simulink model "rlFlyingRobotEnv"  (R2021b)
settings: Solver=VariableStepAuto  StartTime=0.0  StopTime=30  RelTol=1e-3
values from neighbouring files (symbols this model uses):
  theta0 = 0    [main.m]
  Ts = 0.4    [main.m]
  x0 = -15    [main.m]
  y0 = 0    [main.m]
libraries: simulink x3
settings Model: Creator=The MathWorks, Inc.  LastModifiedBy=geek
settings SolverCC: AlgebraicLoopSolver=TrustRegion
settings DataIOCC: ReturnWorkspaceOutputs=off
settings DebuggingCC: SFMachineParentedDataDiag=warning  ArithmeticOperatorsInVariantConditions=warning
settings ModelReferenceCC: ModelReferenceMinAlgLoopOccurrences=on

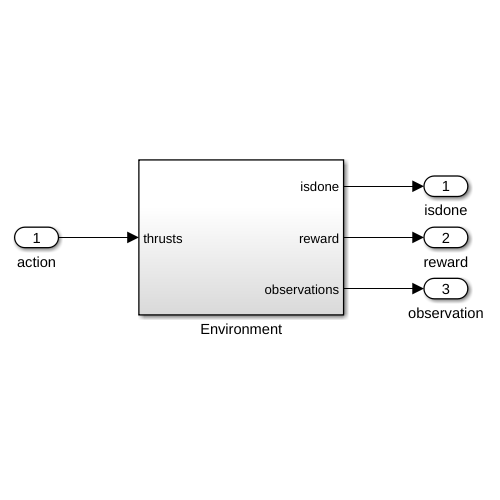
[thumbnail: Simulink's stored preview of the top-level diagram]
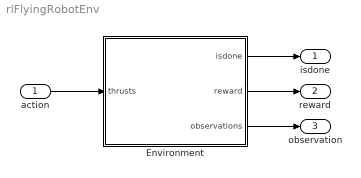
== system rlFlyingRobotEnv ==
  action : Inport
  Environment : Subsystem
  isdone : Outport  VectorParamsAs1DForOutWhenUnconnected=off
  reward : Outport  Port=2  VectorParamsAs1DForOutWhenUnconnected=off
  observation : Outport  Port=3  VectorParamsAs1DForOutWhenUnconnected=off
  wires:
  Environment/3(observations) -> observation/1
  Environment/2(reward) -> reward/1
  Environment/1(isdone) -> isdone/1
  action/1 -> Environment/1(thrusts)

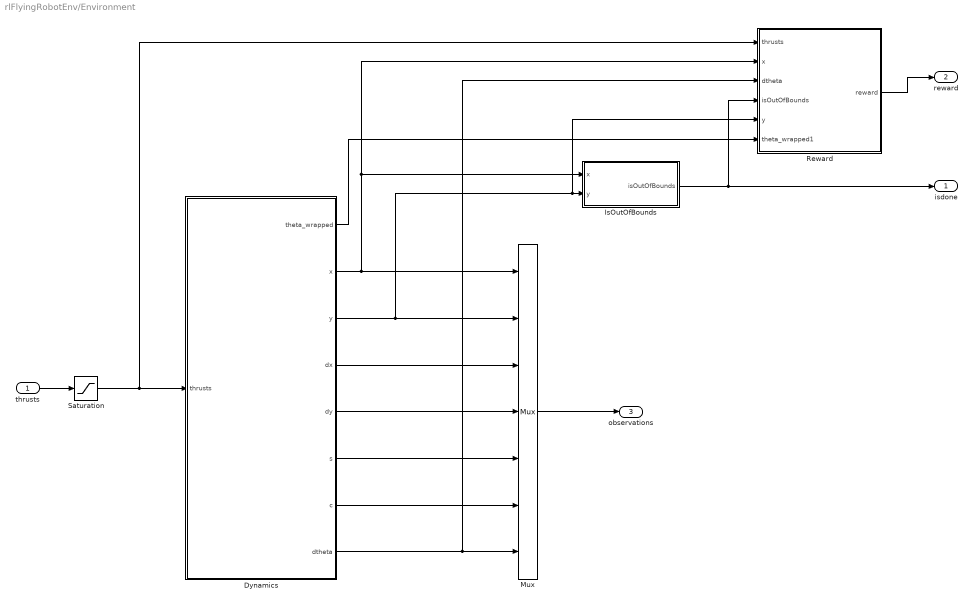
== system rlFlyingRobotEnv/Environment ==
  thrusts : Inport
  Dynamics : Subsystem
  IsOutOfBounds : Subsystem
  Mux : Mux  Inputs=7
  Reward : Subsystem
  Saturation : Saturate  UpperLimit=1  LowerLimit=-1
  isdone : Outport  VectorParamsAs1DForOutWhenUnconnected=off
  reward : Outport  Port=2  VectorParamsAs1DForOutWhenUnconnected=off
  observations : Outport  Port=3  VectorParamsAs1DForOutWhenUnconnected=off
  wires:
  Reward/1(reward) -> reward/1
  IsOutOfBounds/1(isOutOfBounds) -> isdone/1, Reward/4(isOutOfBounds)
  Dynamics/3(y) -> Mux/2, Reward/5(y), IsOutOfBounds/2(y)
  Dynamics/2(x) -> Mux/1, IsOutOfBounds/1(x), Reward/2(x)
  Mux/1 -> observations/1
  Saturation/1 -> Reward/1(thrusts), Dynamics/1(thrusts)
  thrusts/1 -> Saturation/1
  Dynamics/4(dx) -> Mux/3
  Dynamics/5(dy) -> Mux/4
  Dynamics/6(s) -> Mux/5
  Dynamics/7(c) -> Mux/6
  Dynamics/8(dtheta) -> Reward/3(dtheta), Mux/7
  Dynamics/1(theta_wrapped) -> Reward/6(theta_wrapped1)

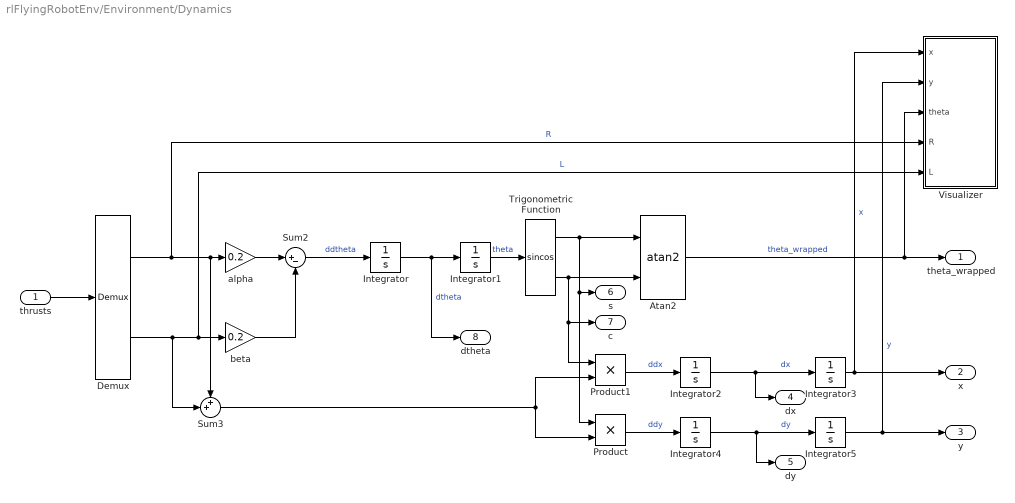
== system rlFlyingRobotEnv/Environment/Dynamics ==
  thrusts : Inport
  Atan2 : Trigonometry  Operator=atan2
  Demux : Demux  Outputs=2
  Integrator : Integrator
  Integrator1 : Integrator  InitialCondition=theta0
  Integrator2 : Integrator
  Integrator3 : Integrator  InitialCondition=x0
  Integrator4 : Integrator
  Integrator5 : Integrator  InitialCondition=y0
  Product : Product
  Product1 : Product
  Sum2 : Sum  Inputs=|+-
  Sum3 : Sum  Inputs=++|
  Trigonometric Function : Trigonometry  Operator=sincos
  Visualizer : Subsystem
  alpha : Gain  Gain=0.2
  beta : Gain  Gain=0.2
  theta_wrapped : Outport  VectorParamsAs1DForOutWhenUnconnected=off
  x : Outport  Port=2  VectorParamsAs1DForOutWhenUnconnected=off
  y : Outport  Port=3  VectorParamsAs1DForOutWhenUnconnected=off
  dx : Outport  Port=4  VectorParamsAs1DForOutWhenUnconnected=off
  dy : Outport  Port=5  VectorParamsAs1DForOutWhenUnconnected=off
  s : Outport  Port=6  VectorParamsAs1DForOutWhenUnconnected=off
  c : Outport  Port=7  VectorParamsAs1DForOutWhenUnconnected=off
  dtheta : Outport  Port=8  VectorParamsAs1DForOutWhenUnconnected=off
  wires:
  Integrator1/1 -> Trigonometric Function/1  "theta"
  Product1/1 -> Integrator2/1  "ddx"
  Integrator2/1 -> dx/1, Integrator3/1  "dx"
  Demux/2 -> Sum3/2, Visualizer/5(L), beta/1  "L"
  Demux/1 -> Visualizer/4(R), Sum3/1, alpha/1  "R"
  Sum3/1 -> Product1/2, Product/2
  Integrator4/1 -> Integrator5/1, dy/1  "dy"
  Trigonometric Function/1 -> s/1, Product/1, Atan2/1
  Trigonometric Function/2 -> Product1/1, c/1, Atan2/2
  Sum2/1 -> Integrator/1  "ddtheta"
  Integrator3/1 -> Visualizer/1(x), x/1  "x"
  Integrator/1 -> dtheta/1, Integrator1/1  "dtheta"
  Product/1 -> Integrator4/1  "ddy"
  Integrator5/1 -> Visualizer/2(y), y/1  "y"
  alpha/1 -> Sum2/1
  beta/1 -> Sum2/2
  thrusts/1 -> Demux/1
  Atan2/1 -> Visualizer/3(theta), theta_wrapped/1  "theta_wrapped"

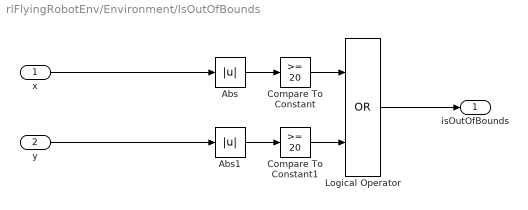
== system rlFlyingRobotEnv/Environment/IsOutOfBounds ==
  x : Inport
  y : Inport  Port=2
  Abs : Abs
  Abs1 : Abs
  Compare To Constant : simulink/Logic and Bit Operations/Compare To Constant  relop=>=  const=20  OutDataTypeStr=boolean
  Compare To Constant1 : simulink/Logic and Bit Operations/Compare To Constant  relop=>=  const=20  OutDataTypeStr=boolean
  Logical Operator : Logic  Operator=OR  AllPortsSameDT=off  OutDataTypeStr=boolean
  isOutOfBounds : Outport  VectorParamsAs1DForOutWhenUnconnected=off
  wires:
  Compare To Constant1/1 -> Logical Operator/2
  Compare To Constant/1 -> Logical Operator/1
  y/1 -> Abs1/1
  Abs/1 -> Compare To Constant/1
  x/1 -> Abs/1
  Abs1/1 -> Compare To Constant1/1
  Logical Operator/1 -> isOutOfBounds/1

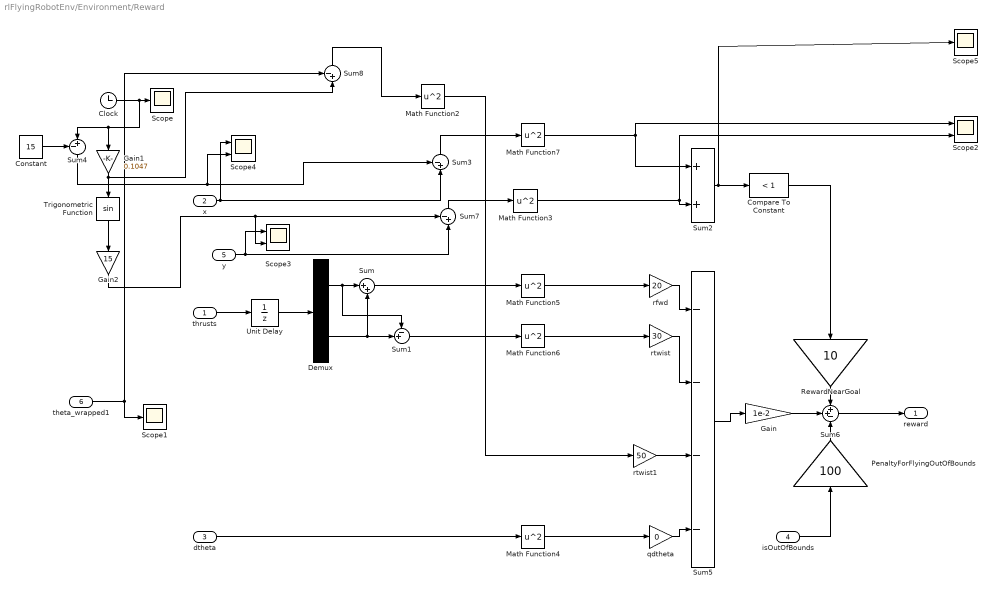
== system rlFlyingRobotEnv/Environment/Reward ==
  thrusts : Inport
  x : Inport  Port=2
  dtheta : Inport  Port=3
  isOutOfBounds : Inport  Port=4
  y : Inport  Port=5
  theta_wrapped1 : Inport  Port=6
  Clock : Clock
      settings: Decimation=30
  Compare To Constant : simulink/Logic and Bit Operations/Compare To Constant  relop=<  const=1  OutDataTypeStr=boolean
  Constant : Constant  Value=15
  Demux : Demux  Outputs=2
  Gain : Gain  Gain=1e-2
  Gain1 : Gain  Gain=0.1047
  Gain2 : Gain  Gain=15
  Math Function{2..7} (6 alike) : Math  Operator=square  SignedPower=on  SaturateOnIntegerOverflow=on
  PenaltyForFlyingOutOfBounds : Gain  Gain=100
  RewardNearGoal : Gain  Gain=10
  Scope : Scope
  Scope1 : Scope
  Scope2 : Scope  NumInputPorts=2
  Scope3 : Scope  NumInputPorts=2
  Scope4 : Scope  NumInputPorts=2
  Scope5 : Scope
  Sum : Sum  Inputs=|++
  Sum{1,3..4,7..8} (5 alike) : Sum  Inputs=-+|
  Sum2 : Sum
  Sum5 : Sum  Inputs=----
  Sum6 : Sum  Inputs=++-
  Trigonometric Function : Trigonometry
  Unit Delay : UnitDelay  SampleTime=Ts  HasFrameUpgradeWarning=on
  qdtheta : Gain  Gain=0
  rfwd : Gain  Gain=20
  rtwist : Gain  Gain=30
  rtwist1 : Gain  Gain=50
  reward : Outport  VectorParamsAs1DForOutWhenUnconnected=off
  wires:
  Sum5/1 -> Gain/1
  thrusts/1 -> Unit Delay/1
  x/1 -> Scope4/1, Sum3/2
  Sum6/1 -> reward/1
  isOutOfBounds/1 -> PenaltyForFlyingOutOfBounds/1
  Unit Delay/1 -> Demux/1
  Demux/1 -> Sum/1, Sum1/1
  Demux/2 -> Sum1/2, Sum/2
  Sum/1 -> Math Function5/1
  Sum1/1 -> Math Function6/1
  Math Function5/1 -> rfwd/1
  Math Function6/1 -> rtwist/1
  qdtheta/1 -> Sum5/4
  Math Function4/1 -> qdtheta/1
  dtheta/1 -> Math Function4/1
  PenaltyForFlyingOutOfBounds/1 -> Sum6/3
  Gain/1 -> Sum6/2
  RewardNearGoal/1 -> Sum6/1
  Compare To Constant/1 -> RewardNearGoal/1
  Sum2/1 -> Scope5/1, Compare To Constant/1
  Clock/1 -> Sum4/2, Gain1/1, Scope/1
  Sum3/1 -> Math Function7/1
  Math Function7/1 -> Scope2/1, Sum2/1
  Constant/1 -> Sum4/1
  Gain1/1 -> Sum8/2, Trigonometric Function/1
  Sum4/1 -> Sum3/1, Scope4/2
  Trigonometric Function/1 -> Gain2/1
  Sum7/1 -> Math Function3/1
  y/1 -> Sum7/2, Scope3/1
  Gain2/1 -> Scope3/2, Sum7/1
  Math Function3/1 -> Sum2/2, Scope2/2
  theta_wrapped1/1 -> Sum8/1, Scope1/1
  Sum8/1 -> Math Function2/1
  rfwd/1 -> Sum5/1
  rtwist/1 -> Sum5/2
  Math Function2/1 -> rtwist1/1
  rtwist1/1 -> Sum5/3

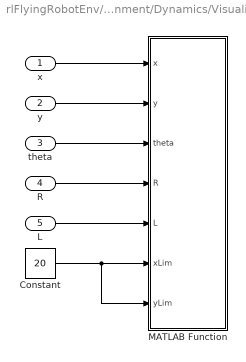
== system rlFlyingRobotEnv/Environment/Dynamics/Visualizer ==
  x : Inport
  y : Inport  Port=2
  theta : Inport  Port=3
  R : Inport  Port=4
  L : Inport  Port=5
  Constant : Constant  Value=20
  MATLAB Function : MATLAB Function  TreatAsAtomicUnit=on
  wires:
  R/1 -> MATLAB Function/4(R)
  y/1 -> MATLAB Function/2(y)
  x/1 -> MATLAB Function/1(x)
  theta/1 -> MATLAB Function/3(theta)
  Constant/1 -> MATLAB Function/7(yLim), MATLAB Function/6(xLim)
  L/1 -> MATLAB Function/5(L)

== matlab function rlFlyingRobotEnv/Environment/Dynamics/Visualizer/MATLAB Function ==
  settings: updateMethod=DISCRETE
  data: x input; y input; theta input; R input; L input; xLim input; yLim input
function fcn(x,y,theta,R,L,xLim,yLim)
%#codegen
coder.extrinsic('rl.env.viz.plotFlyingRobot');
rl.env.viz.plotFlyingRobot(x,y,theta,L,R,xLim,yLim);
